simulink model "GA_tunning_s"  (R2024b)
settings: Solver=ode3  StartTime=0.0  StopTime=1.5*T  FixedStep=1/15  RelTol=1e-3
values from neighbouring files (symbols this model uses):
  a = fzero(sun_syncr, R_E)    [project.m]
  A = [A1 A2 A1 A2 A3 A3]    [project.m]
  A_0 = [-cos(phi) -sin(phi) 0; 0 0 1; -sin(phi) cos(phi) 0]    [project.m]
  A_mis_gyros = eye(3) - [0 -mis_gyros(3) mis_gyros(2); mis_gyros(3) 0 -mis_gyros(1); -mis_gyros(2) mis_gyros(1) 0]    [project.m]
  A_mis_MAG = eye(3) - [0 -mis_MAG(3) mis_MAG(2); mis_MAG(3) 0 -mis_MAG(1); -mis_MAG(2) mis_MAG(1) 0]    [project.m]
  a_S = kep_E(1)    [project.m]
  Acc = 0.75e-2    (= 0.0075)    [project.m]
  alpha = 0.9    [plotPlanet.m]    (also in project.m = [alpha_1 alpha_2]')
  alpha_G_0 = deg2rad(0)    [project.m]
  Area_coil = pi * diameter_coil^2/4    (= 0.000706858347058)    [project.m]
  coil_nominal_resistance = max_voltage_torq^2/power_max_coil    (= 81.6666666667)    [project.m]
  DCM_MIS_SS = eye(3) - [0 -mis_ss(3) mis_ss(2); mis_ss(3) 0 -mis_ss(1); -mis_ss(2) mis_ss(1) 0]    [project.m]
  DCM_SS_B = eye(3)    [project.m]
  e = 0    [project.m]
  e_S = kep_E(2)    [project.m]
  f = 15    [project.m]
  f_mag = 5    [project.m]
  FS_mag = 30    [project.m]
  g = [g1_0 g2_0 g3_0 g4_0 g5_0 g6_0 g7_0 g8_0 g9_0 g10_0  g11_0  g12_0  g13_0 ... (first row only)    [IGRF13_2020.m]
  h = [h1_0 h2_0 h3_0 h4_0 h5_0 h6_0 h7_0 h8_0 h9_0 h10_0  h11_0  h12_0  h13_0 ... (first row only)    [IGRF13_2020.m]
  h_max_RW = 25    [project.m]
  I = diag([Ix_b+Ix_s,Iy_b+Iy_s,Iz_b+Iz_s])    [project.m]
  i = deg2rad(98.3)    [project.m]
  i_S = kep_E(3)    [project.m]
  Izz_RW = 1/2*m_RW*(r_RW^2)    (= 0.12168)    [project.m]
  j_b = 1.4e-3 *[0.2 0.2 1]'*m    [project.m]
  k_filt_g = 0.75    [project.m]
  k_filt_m = 0.75    [project.m]
  k_filt_s = 0.75    [project.m]
  Kb = (1e8)    (= 100000000)    [project.m]
  Lin = 0.015e-2    (= 0.00015)    [project.m]
  linearity_mag_error = 0.02    [project.m]
  max_voltage_torq = 14    [project.m]
  Mounting_error_RW = eye(3) - [0 -mis_RW(3) mis_RW(2); mis_RW(3) 0 -mis_RW(1); -mis_RW(2) mis_RW(1) 0]    [project.m]
  Mounting_matrix_RW = eye(3)    [project.m]
  mu_E = astroConstants(13)    [project.m]
  n = sqrt(mu_E/a^3)    [project.m]
  N_B = [1 0 0; 0 1 0; -1 0 0; 0 -1 0; 0 0 1; 0 0 -1]'    [project.m]
  n_coil = ceil(magnetic_dipole_max/(Area_coil*current_max_coil))    [project.m]
  n_order = 13    [project.m]
  n_S = 2*pi/T_S    [project.m]
  nA_coeff = n_coil*Area_coil    [project.m]
  Noise_Mag = (12e-12)^2    (= 1.44e-22)    [project.m]
  noise_pwm = 50e-6    (= 5e-05)    [project.m]
  Noise_sun_sensor = deg2rad(Acc_ss)^2*t_ss    [project.m]
  OM = deg2rad(270)    [project.m]
  om = 0    [project.m]
  om_0 = [0.08 0.08 0.08]'    [project.m]
  om_detumbling = 4*n    [project.m]
  om_target = [0,0,n]'    [project.m]
  P = Fe/c    [project.m]
  r_F = [l1/2 0 0; 0 l2/2 0; -l1/2 0 0; 0 -l2/2 0; 0 0 (l3+l3_s)/2; 0 0 -(l3+l3_s)/2]'    [project.m]
  R_th = 0.1    [project.m]
  residual_dipole = abs(0.005*magnetic_dipole_max*randn)    [project.m]
  resistance_tol = 0.05*randn    [project.m]
  rho_d = 0.1*ones(6,1)    [project.m]
  rho_S = [0.5, 0.5, 0.5, 0.5, 0.5, 0.1]    [project.m]
  RW_axis = [0;0;1]    [project.m]
  sample_time = 1/f    (= 0.0666666666667)    [project.m]
  sample_time_mag = 1/f_mag    (= 0.2)    [project.m]
  Sens = 100e-6/1e-9    (= 100000)    [project.m]
  Sensor_fov_direction = cos(FS/2)    [project.m]
  Sensor_normal_direction = [0 0 -1]'    [project.m]
  SF_a = 30 * 1e-6    (= 3e-05)    [project.m]
  SF_nl = 30 * 1e-6    (= 3e-05)    [project.m]
  SF_r = 30 * 1e-6    (= 3e-05)    [project.m]
  T_RW_max = 0.2    [project.m]
  t_ss = 1/f_ss    (= 0.2)    [project.m]
  TCR = 0.0039    [project.m]
  th0 = 0    [project.m]
  th_0_S = kep_E(6)    [project.m]
  w0_RW = w_max_RW/4    (= 91.6297857297)    [project.m]
  w_max_RW = 3500*(2*pi)/60    (= 366.519142919)    [project.m]
  w_RW_error = h_RW_error/Izz_RW    (= 0.0164365548981)    [project.m]
undefined symbols (not defined in the file or in its folder): A0, DiscIntNeverNeededParam, K
libraries: matrix_library x15, simulink x4, vrlib x2
(part 2 of 2)

== system GA_tunning_s/Environment/Orbit Definition/Radius of s//c on Earth orbit ==
  Constant1 : Constant  Value=a*(1-e^2)
  Constant2 : Constant  Value=0
  Constant4 : Constant
  Cos : Trigonometry  Operator=cos
  Cos1 : Trigonometry  Operator=cos
  Divide : Product  Inputs=*/
  Eccentricity : Constant  Value=e
  Mux : Mux  Inputs=3
  Perifocal to inertial : Subsystem
  Product1 : Product
  Sin : Trigonometry
  Sum1 : Sum
  True Anomaly : Subsystem
  theta : Outport
  r_direction : Outport  Port=2
  r_magnitude : Outport  Port=3
  theta_dot : Outport  Port=4
  wires:
  Constant4/1 -> Sum1/2
  Cos1/1 -> Product1/2
  Eccentricity/1 -> Product1/1
  Sum1/1 -> Divide/2
  Product1/1 -> Sum1/1
  Divide/1 -> r_magnitude/1  "magnitude of r"
  Cos/1 -> Mux/1
  True Anomaly/1(Theta) -> Cos/1, Sin/1, Cos1/1, theta/1
  Sin/1 -> Mux/2
  Constant1/1 -> Divide/1
  True Anomaly/2(Theta_dot) -> theta_dot/1
  Constant2/1 -> Mux/3
  Perifocal to inertial/1(r_direction) -> r_direction/1
  Mux/1 -> Perifocal to inertial/1(In1)

== system GA_tunning_s/Environment/Orbit Definition/Radius of s//c on Earth orbit wrt Sun ==
  Constant : Constant  Value=[ 1; cos(i_S); sin(i_S)]
  Constant1 : Constant  Value=a_S*(1-e_S^2)
  Constant4 : Constant
  Cos : Trigonometry  Operator=cos
  Cos1 : Trigonometry  Operator=cos
  Divide : Product  Inputs=*/
  Eccentricity : Constant  Value=e
  Mux : Mux  Inputs=3
  Product1 : Product
  Product2 : Product
  Sin : Trigonometry
  Sum1 : Sum
  True Anomaly : Subsystem
  r_Sun_direction : Outport
  r_Sun__magnitude : Outport  Port=2
  wires:
  Sin/1 -> Mux/3, Mux/2
  Sum1/1 -> Divide/2
  Eccentricity/1 -> Product1/1
  Constant4/1 -> Sum1/2
  Cos1/1 -> Product1/2
  Product2/1 -> r_Sun_direction/1
  Mux/1 -> Product2/2
  Divide/1 -> r_Sun__magnitude/1  "magnitude of r_Sun"
  Constant1/1 -> Divide/1
  Cos/1 -> Mux/1
  Constant/1 -> Product2/1
  Product1/1 -> Sum1/1
  True Anomaly/1(Theta_S) -> Cos1/1, Sin/1, Cos/1

== system GA_tunning_s/Environment/SRP/For Each Subsystem ==
  radius : Inport  Partition=on  PartitionDimension=2  PartitionWidth=1  PartitionOffset=0
  Force : Inport  Port=2  Partition=on  PartitionDimension=2  PartitionWidth=1  PartitionOffset=0
  Cross Product : vrlib/Utilities/Cross Product
  For Each : ForEach  DisableCoverage=on
  Out1 : Outport  ConcatenationDimension=2
  wires:
  radius/1 -> Cross Product/1
  Force/1 -> Cross Product/2
  Cross Product/1 -> Out1/1

== system GA_tunning_s/Environment/SRP/For Each Subsystem1 ==
  In1 : Inport  Partition=on  PartitionDimension=2  PartitionWidth=1  PartitionOffset=0
  Constant : Constant  Value=0
  For Each : ForEach  DisableCoverage=on
  Switch : Switch  Criteria=u2 > Threshold  SaturateOnIntegerOverflow=off  InputSameDT=off
  Out1 : Outport  ConcatenationDimension=2
  wires:
  In1/1 -> Switch/1, Switch/2
  Constant/1 -> Switch/3
  Switch/1 -> Out1/1

== system GA_tunning_s/Environment/SRP/Norm ==
  In1 : Inport
  Dot Product : DotProduct  OutDataTypeStr=Inherit: Inherit via internal rule
  Square Root : Sqrt
  Out1 : Outport
  wires:
  Square Root/1 -> Out1/1
  In1/1 -> Dot Product/2, Dot Product/1
  Dot Product/1 -> Square Root/1

== system GA_tunning_s/Kinematics/Matrix A_BN/Orthonormalization of A(t) ==
  A(t) : Inport
  Gain : Gain  Gain=1/2
  Gain1 : Gain  Gain=3/2
  Product1 : Product  Inputs=3  Multiplication=Matrix(*)
  Sum : Sum  Inputs=|+-
  Transpose : Math  Operator=transpose
  A(t) orthonormal : Outport
  wires:
  A(t)/1 -> Product1/3, Gain1/1, Gain/1, Transpose/1
  Transpose/1 -> Product1/2
  Product1/1 -> Sum/2
  Gain1/1 -> Sum/1
  Gain/1 -> Product1/1
  Sum/1 -> A(t) orthonormal/1

== system GA_tunning_s/Sensors/Gyro/Filter ==
  Input : Inport
  Delay1 : Delay  DelayLength=1  InitialConditionSource=Input port  SampleTime=t_ss
      settings: InputPortMap=u0,p4
  Gain : Gain  Gain=1-k_filt_g
  Gain1 : Gain  Gain=k_filt_g
  Sum1 : Sum  Inputs=|++
  Output : Outport
  wires:
  Input/1 -> Delay1/2, Gain/1
  Sum1/1 -> Delay1/1, Output/1
  Gain/1 -> Sum1/2
  Gain1/1 -> Sum1/1
  Delay1/1 -> Gain1/1

== system GA_tunning_s/Sensors/Magnetometer/Filter ==
  Input : Inport
  Delay1 : Delay  DelayLength=1  InitialConditionSource=Input port  SampleTime=sample_time_mag
      settings: InputPortMap=u0,p4
  Gain : Gain  Gain=1-k_filt_m
  Gain1 : Gain  Gain=k_filt_m
  Sum1 : Sum  Inputs=|++
  Output : Outport
  wires:
  Input/1 -> Delay1/2, Gain/1
  Sum1/1 -> Delay1/1, Output/1
  Gain/1 -> Sum1/2
  Gain1/1 -> Sum1/1
  Delay1/1 -> Gain1/1

== system GA_tunning_s/Sensors/Sun sensor/Filter ==
  Input : Inport
  Delay1 : Delay  DelayLength=1  InitialConditionSource=Input port  SampleTime=t_ss
      settings: InputPortMap=u0,p4
  Gain : Gain  Gain=1-k_filt_s
  Gain1 : Gain  Gain=k_filt_s
  Sum1 : Sum  Inputs=|++
  Output : Outport
  wires:
  Input/1 -> Delay1/2, Gain/1
  Sum1/1 -> Delay1/1, Output/1
  Gain/1 -> Sum1/2
  Gain1/1 -> Sum1/1
  Delay1/1 -> Gain1/1

== system GA_tunning_s/Sensors/Sun sensor/Unit vector ==
  Sun vector : Inport
  Divide : Product  Inputs=*/
  Dot Product : DotProduct  OutDataTypeStr=Inherit: Inherit via internal rule
  Sqrt : Sqrt
  Out1 : Outport
  wires:
  Dot Product/1 -> Sqrt/1
  Divide/1 -> Out1/1
  Sun vector/1 -> Divide/1, Dot Product/2, Dot Product/1
  Sqrt/1 -> Divide/2

== system GA_tunning_s/Attitude Determination/Attitude determination kinematic method/Matrix A_BN/Orthonormalization of A(t)1 ==
  A(t) : Inport
  Gain : Gain  Gain=1/2
  Gain1 : Gain  Gain=3/2
  Product1 : Product  Inputs=3  Multiplication=Matrix(*)
  Sum : Sum  Inputs=|+-
  Transpose : Math  Operator=transpose
  A(t) orthonormal : Outport
  wires:
  Sum/1 -> A(t) orthonormal/1
  Gain/1 -> Product1/1
  Gain1/1 -> Sum/1
  Product1/1 -> Sum/2
  Transpose/1 -> Product1/2
  A(t)/1 -> Transpose/1, Gain/1, Gain1/1, Product1/3

== system GA_tunning_s/Environment/Orbit Definition/Radius of s//c on Earth orbit/Perifocal to inertial ==
  In1 : Inport
  Constant : Constant  Value=[1 0 0; 0 cos(i) sin(i); 0 -sin(i) cos(i)]
  Constant1 : Constant  Value=[cos(OM) sin(OM) 0; -sin(OM) cos(OM) 0; 0 0 1]
  Constant2 : Constant  Value=[cos(om) sin(om) 0; -sin(om) cos(om) 0; 0 0 1]
  MatrixMultiply : Product  Multiplication=Matrix(*)
  Product : Product  Inputs=3  Multiplication=Matrix(*)
  Transpose : Math  Operator=transpose
  Transpose1 : Math  Operator=transpose
  Transpose2 : Math  Operator=transpose
  r_direction : Outport
  wires:
  Constant/1 -> Transpose/1
  Constant1/1 -> Transpose1/1
  Constant2/1 -> Transpose2/1
  Transpose1/1 -> Product/1
  Transpose/1 -> Product/2
  Transpose2/1 -> Product/3
  Product/1 -> MatrixMultiply/1
  In1/1 -> MatrixMultiply/2
  MatrixMultiply/1 -> r_direction/1

== system GA_tunning_s/Environment/Orbit Definition/Radius of s//c on Earth orbit/True Anomaly ==
  Constant : Constant  Value=th0
  Constant3 : Constant
  Cos : Trigonometry  Operator=cos
  Gain : Gain  Gain=n/(1-e^2)^(3/2)
  Gain1 : Gain  Gain=e
  Integrator : Integrator  InitialConditionSource=external  WrapState=on  WrappedStateUpperValue=2*pi  WrappedStateLowerValue=0
  Square : Math  Operator=square
  Sum : Sum
  To Workspace : ToWorkspace  VariableName=theta  SampleTime=-1
  Theta : Outport
  Theta_dot : Outport  Port=2
  wires:
  Gain1/1 -> Sum/2
  Constant3/1 -> Sum/1
  Cos/1 -> Gain1/1
  Integrator/1 -> To Workspace/1, Theta/1, Cos/1  "theta"
  Sum/1 -> Square/1
  Constant/1 -> Integrator/2
  Square/1 -> Gain/1
  Gain/1 -> Theta_dot/1, Integrator/1

== system GA_tunning_s/Environment/Orbit Definition/Radius of s//c on Earth orbit wrt Sun/True Anomaly ==
  Constant : Constant  Value=th_0_S
  Constant3 : Constant
  Cos : Trigonometry  Operator=cos
  Gain : Gain  Gain=n_S/(1-e_S^2)^(3/2)
  Gain1 : Gain  Gain=e_S
  Integrator : Integrator  InitialConditionSource=external  WrapState=on  WrappedStateUpperValue=2*pi  WrappedStateLowerValue=0
  Square : Math  Operator=square
  Sum : Sum
  To Workspace : ToWorkspace  VariableName=theta_S  SampleTime=-1
  Theta_S : Outport
  wires:
  Gain1/1 -> Sum/2
  Constant3/1 -> Sum/1
  Cos/1 -> Gain1/1
  Integrator/1 -> To Workspace/1, Theta_S/1, Cos/1  "theta"
  Sum/1 -> Square/1
  Constant/1 -> Integrator/2
  Square/1 -> Gain/1
  Gain/1 -> Integrator/1

== matlab function GA_tunning_s/Environment/Magnetic Torque/MATLAB Function ==
  data: r_n input; B_N output; t input; g input; h input; alpha_G_0 input; n_order input
function B_N  = Earth_mag_field(r_n, t, g, h, alpha_G_0, n_order)

%  Earth's Magnetic Field using spherical harmonics until order 13.
%Gaussian Coefficients from IGRF  2020 
%
%--------------------------------------------------------------------------
% INPUTS:
%   r_n            S/C Position in inertial frame [km]
%   t              Time [s]
%   g              g_nm Matrix   [T]
%   h              h_nm Matrix   [T]
%   alpha_G_0      Greenwich Longitude [rad]
%   n              Order [-]
% --------------------------------------------------------------------------
% OUTPUTS:
%   B_N            Magnetic field   [T]
% --------------------------------------------------------------------------
% References :Lecture_notes_prof_Bernelli_part1


%% Pre-Settings 

S_nm = zeros(n_order+1,n_order);
S_00 = 1;

P_nm = zeros(n_order+1,n_order);
P_00 = 1;

d_P_nm = zeros(n_order+1,n_order);
d_P_00 = 0;

K_nm = zeros(n_order+1,n_order);

g_nm = zeros(n_order+1,n_order);
h_nm = zeros(n_order+1,n_order);

%% Topocentric Horizon Angles
x = r_n(1,1);
y = r_n(2,1);
z = r_n(3,1);

r_norm = norm(r_n);

% Earth Radius [km]
Re = 6371.2;

% Earth Angular Velocity [rad/sec]
om_E = 7.292124*1e-5;

% Declination ( Latitude )
delta = asin(z/r_norm);

% Coelevation
theta = pi/2 - delta;

% Greenwich Meridian Longitude
alpha_G = alpha_G_0 + t * om_E;

% Right Ascension (Local Sidereal Time)
if (y/r_norm) > 0
    alpha = acos((x/r_norm)/cos(delta));
else
    alpha = 2*pi - acos((x/r_norm)/cos(delta));
end

% Longitude
phi = alpha - alpha_G;

%% Gauss Normalization
for j = 1 : n_order
    if j == 1
        S_nm(1,j) = S_00 * ((2*j - 1)/j);
    elseif j >= 2
        S_nm(1,j) = S_nm(1,j-1)*((2*j - 1)/j);
    end
end
%Remaining Components (S_n,m)
for j = 1 : n_order
    for i = 2 : j+1
            S_nm(i,j) = S_nm(i-1,j)*sqrt(((kronDel(1,i-1) + 1)*(j - (i-1) + 1))...
                                    /(j + (i -1)));
    end
end

%Coefficients K^n,m
for j = 1 : n_order
    for i = 1 : j+1
        if j == 1
            K_nm(i,j) = 0;
        elseif j > 1
            K_nm(i,j) = ((j - 1)^2 - (i-1)^2) / ((2*j - 1)*(2*j - 3));
        end
    end
end

% P^n,m
P_nm(1,1) = cos(theta)*P_00;        %P_1,0
P_nm(2,1) = sin(theta)*P_00;        %P_1,1
for j = 2 : n_order
    for i = 1 : j+1
        if i-1 == j                             %P_n,n
            P_nm(i,j) = sin(theta)*P_nm(j,j-1);
        else
            if j < 3                            %P_n,m
                P_nm(i,j) = cos(theta)*P_nm(i,j-1);
            else
                P_nm(i,j) = cos(theta)*P_nm(i,j-1) - K_nm(i,j)*P_nm(i,j-2);
            end
        end
    end
end

% d_P^n,m (wrt theta)
d_P_nm(1,1) = cos(theta)*d_P_00 - sin(theta)*P_00; %d_P_1,0
d_P_nm(2,1) = sin(theta)*d_P_00 + cos(theta)*P_00; %d_P_1,1
for j = 2 : n_order
    for i = 1 : j+1
        if i-1 == j
            d_P_nm(i,j) = sin(theta)*d_P_nm(j,j-1) + cos(theta)*P_nm(j,j-1);
        else
            if j < 3
                d_P_nm(i,j) = cos(theta)*d_P_nm(i,j-1) - sin(theta)*P_nm(i,j-1);
            else
                d_P_nm(i,j) = cos(theta)*d_P_nm(i,j-1) - ...
                        sin(theta)*P_nm(i,j-1) - K_nm(i,j)*d_P_nm(i,j-2);
            end
        end
    end
end

%% Guassian Coefficients Normalization

for j = 1 : n_order
    for i = 1 : j+1
        g_nm(i,j) = S_nm(i,j)*g(i,j);
        h_nm(i,j) = S_nm(i,j)*h(i,j);
    end
end

%% Magnetic Field Components - Spherical Coordinates

%Reset Handle Variables
dx = 0;
pr = 0;
%Radial Component
for j = 1 : n_order
    sx = (Re/norm(r_n))^(j+2) * (j + 1);
    for i = 1 : j+1
        dx = dx + (g_nm(i,j)*cos((i-1)*phi) + h_nm(i,j)*sin((i-1)*phi)) * P_nm(i,j);
    end
    pr = pr + sx*dx;
    dx = 0;
end
B_r = pr;

%Reset Handle Variables
dx = 0;
pr = 0;
%Coelevation Component
for j = 1 : n_order
    sx = ((Re/norm(r_n))^(j+2));
    for i = 1 : j+1
        dx = dx + (g_nm(i,j)*cos((i-1)*phi) + h_nm(i,j)*sin((i-1)*phi)) * d_P_nm(i,j);
    end
    pr = pr + sx*dx;
    dx = 0;
end
B_th = -pr;

%Reset Handle Variables
dx = 0;
pr = 0;
%Azimuth Component
for j = 1 : n_order
    sx = ((Re/norm(r_n))^(j+2));
    for i = 1 : j+1
        dx = dx + (i*(-g_nm(i,j)*sin((i-1)*phi) + h_nm(i,j)*cos((i-1)*phi)) * P_nm(i,j));
    end
    pr = pr + sx*dx;
    dx = 0;
end
B_phi = -1/sin(theta) * pr;

%% Magnetic Field Components - Inertial Ref. Frame

B_1 = (B_r*cos(delta) + B_th*sin(delta))*cos(alpha) - B_phi*sin(alpha);
B_2 = (B_r*cos(delta) + B_th*sin(delta))*sin(alpha) + B_phi*cos(alpha);
B_3 = (B_r*sin(delta) - B_th*cos(delta));
B_N = [B_1; B_2; B_3];

end

%% Kronecker Delta Function

function d = kronDel(j,k)
if j == k
    d = 1;
else
    d = 0;
end
end

== matlab function GA_tunning_s/Attitude Determination/Attitude determination Wabha problem /SVD ==
  data: B input; U output; M output; V_T output
function[U,M,V_T] = svd(B)

[U,~,V]=svd(B);
M = diag([1 1 det(U)*det(V)]);
V_T = V';

end
